simulink library "Chassis_Alpha_sm_s3d_org"  (Simulink 10.0)
settings: Solver=ode45  StartTime=0.0  StopTime=10.0  RelTol=1e-3  EnableMultiTasking=on
undefined symbols (not defined in the file): Chassis, open_system
libraries: Chassis_Alpha x2, Chassis_Alpha_sm x1, vrlib x1, simulink x1
Description:
  | Copyright 2013-2014 The MathWorks, Inc.
settings Model: Creator=mbrauer  LastModifiedBy=annonymous

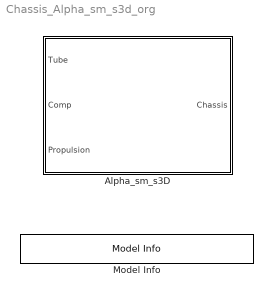
== system Chassis_Alpha_sm_s3d_org ==
  Alpha_sm_s3D : Subsystem  InitFcn=open_system([gcb,'/VR Sink'])
  Model Info : simulink/Model-Wide Utilities/Model Info  Frame=on  DisplayStringWithTags=%<Description>  HorizontalTextAlignment=Center  LeftAlignmentValue=0.5

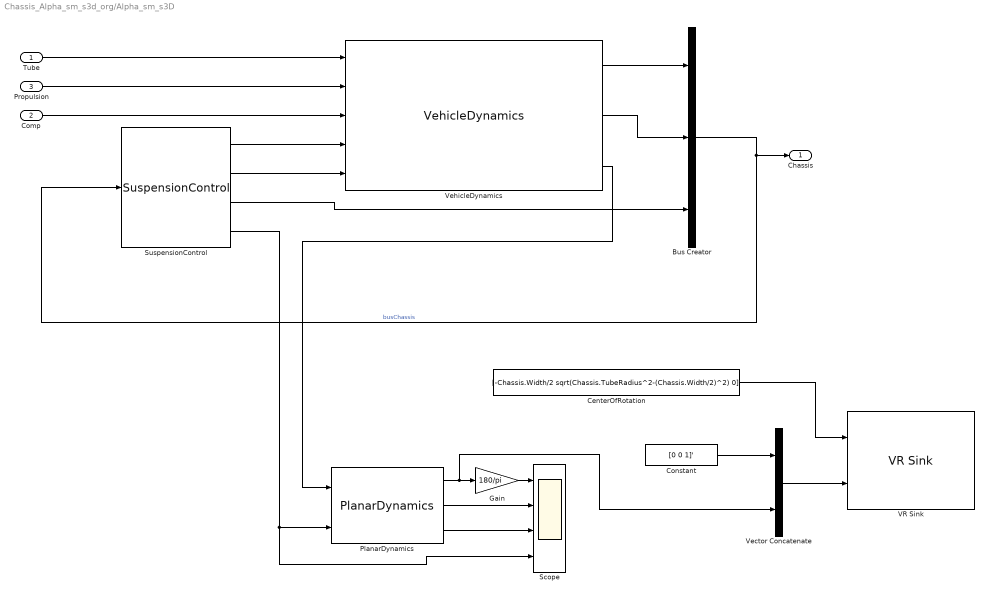
== system Chassis_Alpha_sm_s3d_org/Alpha_sm_s3D ==
  "Tube " : Inport
  Comp : Inport  Port=2
  Propulsion : Inport  Port=3
  Bus Creator : BusCreator  Inputs=3  NonVirtualBus=on
  CenterOfRotation : Constant  Value=[-Chassis.Width/2 sqrt(Chassis.TubeRadius^2-(Chassis.Width/2)^2) 0]'
  Constant : Constant  Value=[0 0 1]'
  Gain : Gain  Gain=180/pi
  PlanarDynamics : Chassis_Alpha_sm/PlanarDynamics  R=Chassis.TubeRadius  cH=Chassis.Height  cW=Chassis.Width  M=Chassis.Mass  D=5e3 % magic number
  Scope : Scope  NumInputPorts=4
  SuspensionControl : Chassis_Alpha/SuspensionControl
  VR Sink : vrlib/VR Sink  InstantiateOnLoad=on  SampleTime=0.1  ViewEnable=on  RemoteChange=off  RemoteView=off  FieldsWritten=HyperPod.center.3.1.1.double#HyperPod.rotation.4.1.1.double  WorldFileName=hyperLoopPod3D.wrl  AutoView=off  VideoDimensions=[]  AllowVariableSize=off
      settings: SourceProductName=Simulink
  Vector Concatenate : Concatenate
  VehicleDynamics : Chassis_Alpha/VehicleDynamics
  Chassis : Outport
  wires:
  Gain/1 -> Scope/1
  VehicleDynamics/3 -> PlanarDynamics/1
  SuspensionControl/4 -> PlanarDynamics/2, Scope/4
  PlanarDynamics/3 -> Scope/3
  PlanarDynamics/2 -> Scope/2
  Vector Concatenate/1 -> VR Sink/2
  CenterOfRotation/1 -> VR Sink/1
  Constant/1 -> Vector Concatenate/1
  PlanarDynamics/1 -> Vector Concatenate/2, Gain/1
  Bus Creator/1 -> SuspensionControl/1, Chassis/1  "busChassis"
  Comp/1 -> VehicleDynamics/3
  "Tube "/1 -> VehicleDynamics/1
  VehicleDynamics/1 -> Bus Creator/1
  VehicleDynamics/2 -> Bus Creator/2
  Propulsion/1 -> VehicleDynamics/2
  SuspensionControl/1 -> VehicleDynamics/4
  SuspensionControl/2 -> VehicleDynamics/5
  SuspensionControl/3 -> Bus Creator/3
